simulink model "qiwanghengbai"  (R2024b)
settings: Solver=VariableStepAuto  StartTime=0.0  StopTime=10.0  RelTol=1e-3
values from neighbouring files (symbols this model uses):
  g = 9.8    [nihe.m]    (also in nihecepiangangducfcr.m)
  k = m/L*(b/Kf-a/Kr)    (= 0.000236258958887)    [canshu.m]
  L = a+b    (= 2.05)    [canshu.m]
  v = 108/3.6    (= 30)    [canshu.m]
libraries: Solver_SF x1
settings Model: Creator=28677  LastModifiedBy=28677

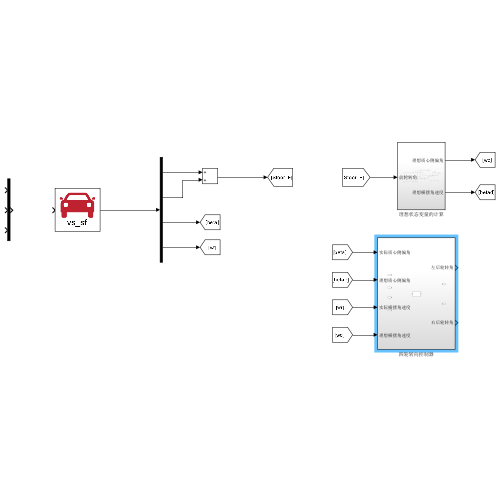
[thumbnail: Simulink's stored preview of the top-level diagram]
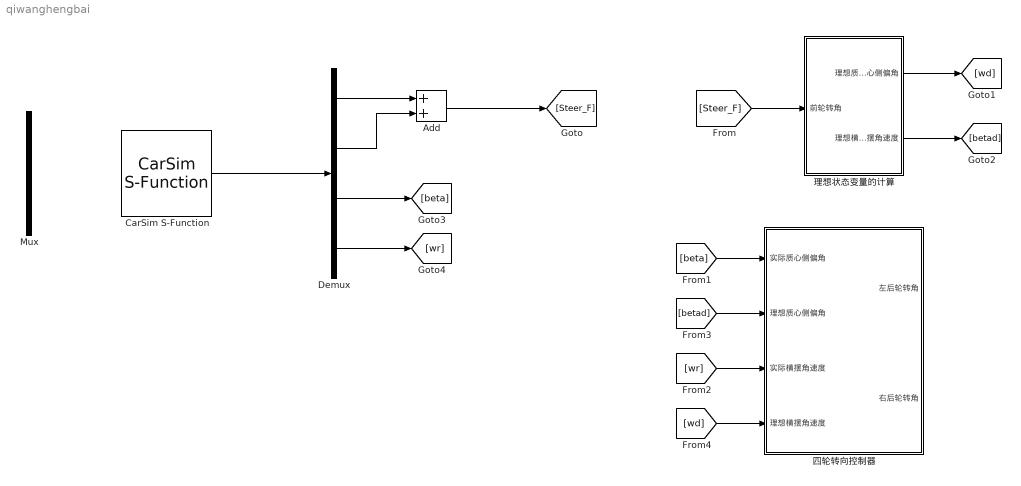
== system qiwanghengbai ==
  Add : Sum
  CarSim S-Function : Solver_SF/CarSim S-Function  Priority=1  SIMFILE=simfile.sim  Run_RTs=off  vs_state_ind=Run  StopMode_ind=Vehicle Model
  Demux : Demux
  Mux : Mux  Inputs=3
  四轮转向控制器 : Subsystem
  理想状态变量的计算 : Subsystem
  wires:
  CarSim S-Function/1 -> Demux/1
  Demux/1 -> Add/1
  Demux/2 -> Add/2
  Add/1 -> [Steer_F]
  [Steer_F] -> 理想状态变量的计算/1(前轮转角)
  理想状态变量的计算/1(理想质心侧偏角) -> [wd]
  理想状态变量的计算/2(理想横摆角速度) -> [betad]
  Demux/3 -> [beta]
  Demux/4 -> [wr]
  [beta] -> 四轮转向控制器/1(实际质心侧偏角)
  [wr] -> 四轮转向控制器/3(实际横摆角速度)
  [betad] -> 四轮转向控制器/2(理想质心侧偏角)
  [wd] -> 四轮转向控制器/4(理想横摆角速度)

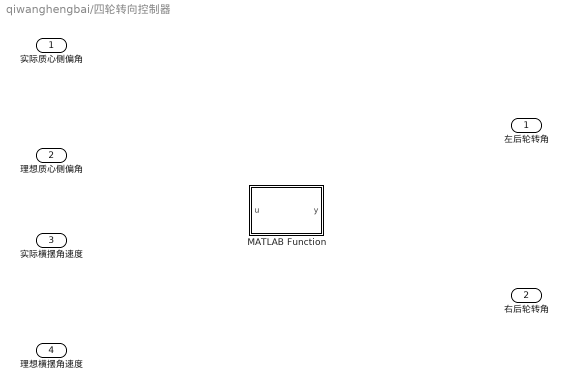
== system qiwanghengbai/四轮转向控制器 ==
  实际质心侧偏角 : Inport
  理想质心侧偏角 : Inport  Port=2
  实际横摆角速度 : Inport  Port=3
  理想横摆角速度 : Inport  Port=4
  MATLAB Function : MATLAB Function  TreatAsAtomicUnit=on
  左后轮转角 : Outport
  右后轮转角 : Outport  Port=2

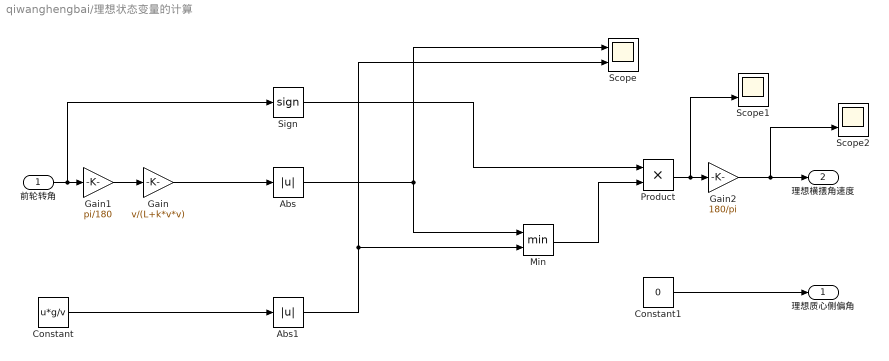
== system qiwanghengbai/理想状态变量的计算 ==
  前轮转角 : Inport
  Abs : Abs  SaturateOnIntegerOverflow=off
  Abs1 : Abs  SaturateOnIntegerOverflow=off
  Constant : Constant  Value=u*g/v
  Constant1 : Constant  Value=0
  Gain : Gain  Gain=v/(L+k*v*v)
  Gain1 : Gain  Gain=pi/180
  Gain2 : Gain  Gain=180/pi
  Min : MinMax  Inputs=2
  Product : Product
  Scope : Scope  NumInputPorts=2
  Scope1 : Scope  NumInputPorts=2
  Scope2 : Scope  NumInputPorts=2
  Sign : Signum
  理想质心侧偏角 : Outport
  理想横摆角速度 : Outport  Port=2
  wires:
  前轮转角/1 -> Sign/1, Gain1/1
  Gain1/1 -> Gain/1
  Gain/1 -> Abs/1
  Constant/1 -> Abs1/1
  Abs/1 -> Min/1, Scope/1
  Abs1/1 -> Scope/2, Min/2
  Sign/1 -> Product/1
  Min/1 -> Product/2
  Product/1 -> Scope1/2, Gain2/1
  Constant1/1 -> 理想质心侧偏角/1
  Gain2/1 -> Scope2/2, 理想横摆角速度/1

== matlab function qiwanghengbai/四轮转向控制器/MATLAB Function ==
  data: u input; y output
function y = fcn(u)

y = u;
